simulink model "lab2_task3"  (R2020a)
settings: Solver=FixedStepDiscrete  StartTime=0.0  StopTime=inf  FixedStep=0.02  RelTol=1e-3  EnableMultiTasking=on
values from neighbouring files (symbols this model uses):
  lim = length(xx)    [lab2_task3_4_trajectories.m]
  tt = zeros(size(xx))    [lab2_task3_4_trajectories.m]
  xx = 0:0.5:2*3.14    [lab2_task3_4_trajectories.m]
  yy = sin(0:0.5:2*3.14)    [lab2_task3_4_trajectories.m]
undefined symbols (not defined in the file or in its folder): angdiff, Angular, Linear
libraries: robotlib x3, simulink x2, robotcorelib x1, simulink_extras x1
settings Model: Creator=The MathWorks, Inc.  LastModifiedBy=Pablo
settings DataIOCC: LimitDataPoints=on  SaveFormat=Array  ReturnWorkspaceOutputs=off
settings OptimizationCC: ZeroExternalMemoryAtStartup=off  ZeroInternalMemoryAtStartup=off  LifeSpan=Inf  MaxStackSize=64
settings DebuggingCC: SolverPrmCheckMsg=warning  AllowSymbolicDim=off  SFUnexpectedBacktrackingDiag=warning  SFNoUnconditionalDefaultTransitionDiag=warning  SFExecutionAtInitializationDiag=none  ArithmeticOperatorsInVariantConditions=warning
settings HardwareCC: ProdBitPerPointer=32  ProdBitPerSizeT=32  ProdBitPerPtrDiffT=32  ProdLargestAtomicFloat=None  ProdIntDivRoundTo=Undefined  ProdEndianess=Unspecified  ProdWordSize=32  ProdHWDeviceType=Generic->Unspecified (assume 32-bit Generic)  TargetHWDeviceType=Generic->Unspecified (assume 32-bit Generic)  UseEmbeddedCoderFeatures=off
settings ModelReferenceCC: PropagateSignalLabelsOutOfModel=off
settings SFSimCC: SimUseLocalCustomCode=off  CustomCodeUndefinedFunction=UseInterfaceOnly
settings RTWCC: SystemTargetFile=ert.tlc  HardwareBoard=Robot Operating System (ROS)  TemplateMakefile=ert_default_tmf  RTWUseLocalCustomCode=off  Toolchain=Catkin  TargetLang=C++
settings CodeAppCC: StateflowObjectComments=on
settings ERTTargetCC: MultiwordLength=2048  ERTCustomFileBanners=off  MultiInstanceERTCode=on  CodeInterfacePackaging=C++ class  SupportContinuousTime=on  SupportNonInlinedSFcns=on  RemoveResetFunc=off  SupportVariableSizeSignals=on  ModelStepFunctionPrototypeControlCompliant=off  RootIOFormat=Structure reference  ConvertIfToSwitch=off  SuppressUnreachableDefaultCases=off
settings ConfigComp: CovMetricSettings=dw  CovHtmlReporting=on  CovSaveCumulativeToWorkspaceVar=on  CovSaveSingleToWorkspaceVar=on  CovExternalEMLEnable=off  CovSFcnEnable=off

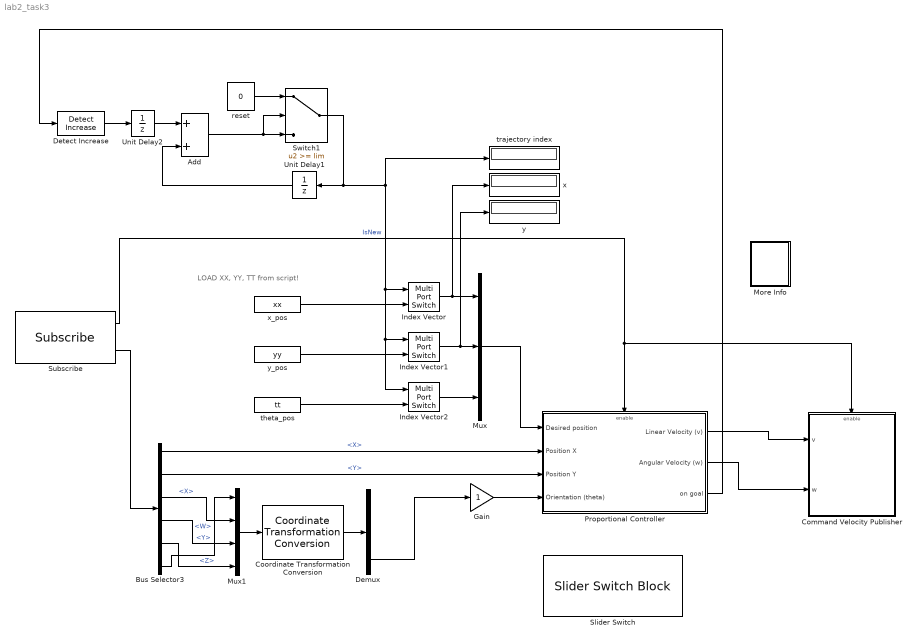
== system lab2_task3 ==
  note: LOAD XX, YY, TT from script!
  Add : Sum
  Bus Selector3 : BusSelector  OutputSignals=Pose.Pose.Position.X,Pose.Pose.Position.Y,Pose.Pose.Orientation.X,Pose.Pose.Orientation.Y,Pose.Pose.Orientation.Z,Pose.Pose.Orientation.W
  Command Velocity Publisher : Subsystem
  Coordinate Transformation Conversion : robotcorelib/Coordinate Transformation Conversion  InputRepresentation=Quaternion  InputEulerSequence=XYZ  ShowTrVecInputPort=on  OutputRepresentation=Euler Angles  OutputEulerSequence=XYZ  ShowTrVecOutputPort=on  SimulateUsing=Interpreted execution
      settings: SourceProductBaseCode=NV,RO,RR
  Demux : Demux  Outputs=3
  Detect Increase : simulink/Logic and Bit Operations/Detect Increase  vinit=0.0  OutDataTypeStr=boolean
  Gain : Gain
  Index Vector : MultiPortSwitch  DataPortOrder=Zero-based contiguous  Inputs=1  zeroidx=on
  Index Vector1 : MultiPortSwitch  DataPortOrder=Zero-based contiguous  Inputs=1  zeroidx=on
  Index Vector2 : MultiPortSwitch  DataPortOrder=Zero-based contiguous  Inputs=1  zeroidx=on
  More Info : Subsystem
      settings: OpenFcn=showdemo(bdroot(gcb))
      mask Display: disp('?')
  Mux : Mux  Inputs=3
  Mux1 : Mux
  Proportional Controller : Subsystem
  Slider Switch : SliderSwitchBlock
      settings: Values={{'STOP OFF', 'STOP ON'}, [0 1]}
  Subscribe : robotlib/Subscribe  topicSource=Select from ROS network  topic=/odom  messageType=nav_msgs/Odometry  sampleTime=-1  messageQueueLength=51
  Switch1 : Switch  Threshold=lim
  Unit Delay1 : UnitDelay  SampleTime=-1  HasFrameUpgradeWarning=on
  Unit Delay2 : UnitDelay  SampleTime=-1  HasFrameUpgradeWarning=on
  reset : Constant  Value=0  VectorParams1D=off
  theta_pos : Constant  Value=tt  VectorParams1D=off
  trajectory index : Display
  x : Display
  x_pos : Constant  Value=xx  VectorParams1D=off
  y : Display
  y_pos : Constant  Value=yy  VectorParams1D=off
  wires:
  Subscribe/2 -> Bus Selector3/1
  Subscribe/1 -> Command Velocity Publisher/Enable, Proportional Controller/Enable  "IsNew"
  Mux/1 -> Proportional Controller/1(Desired position)
  Mux1/1 -> Coordinate Transformation Conversion/1
  Coordinate Transformation Conversion/1 -> Demux/1
  Proportional Controller/2(Angular Velocity (w)) -> Command Velocity Publisher/2(w)
  Proportional Controller/1(Linear Velocity (v)) -> Command Velocity Publisher/1(v)
  Bus Selector3/1 -> Proportional Controller/2(Position X)  "<X>"
  Bus Selector3/2 -> Proportional Controller/3(Position Y)  "<Y>"
  Gain/1 -> Proportional Controller/4(Orientation (theta))
  Bus Selector3/3 -> Mux1/2  "<X>"
  Bus Selector3/4 -> Mux1/3  "<Y>"
  Bus Selector3/5 -> Mux1/4  "<Z>"
  Bus Selector3/6 -> Mux1/1  "<W>"
  Demux/3 -> Gain/1
  Add/1 -> Switch1/2, Switch1/3
  Unit Delay1/1 -> Add/2
  reset/1 -> Switch1/1
  Index Vector2/1 -> Mux/3
  Index Vector1/1 -> y/1, Mux/2
  Index Vector/1 -> Mux/1, x/1
  x_pos/1 -> Index Vector/2
  y_pos/1 -> Index Vector1/2
  theta_pos/1 -> Index Vector2/2
  Proportional Controller/3(on goal) -> Detect Increase/1
  Detect Increase/1 -> Unit Delay2/1
  Unit Delay2/1 -> Add/1
  Switch1/1 -> trajectory index/1, Index Vector1/1, Index Vector2/1, Index Vector/1, Unit Delay1/1

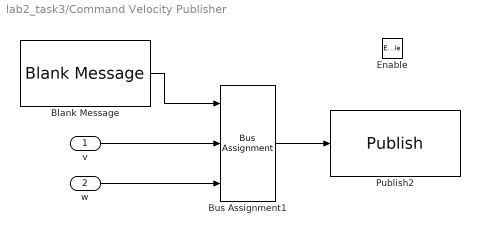
== system lab2_task3/Command Velocity Publisher ==
  v : Inport
  w : Inport  Port=2
  Enable : EnablePort
  Blank Message : robotlib/Blank Message  messageClass=Message  entityType=geometry_msgs/Twist  messageType=geometry_msgs/Twist  SampleTime=inf
  Bus Assignment1 : BusAssignment  DialogController=Simulink.DDGSource_BusAssignment  AssignedSignals=Linear.X,Angular.Z
  Publish2 : robotlib/Publish  topicSource=Select from ROS network  topic=/cmd_vel  messageType=geometry_msgs/Twist  messageQueueLength=105
  wires:
  Bus Assignment1/1 -> Publish2/1
  Blank Message/1 -> Bus Assignment1/1
  v/1 -> Bus Assignment1/2
  w/1 -> Bus Assignment1/3

== system lab2_task3/More Info ==

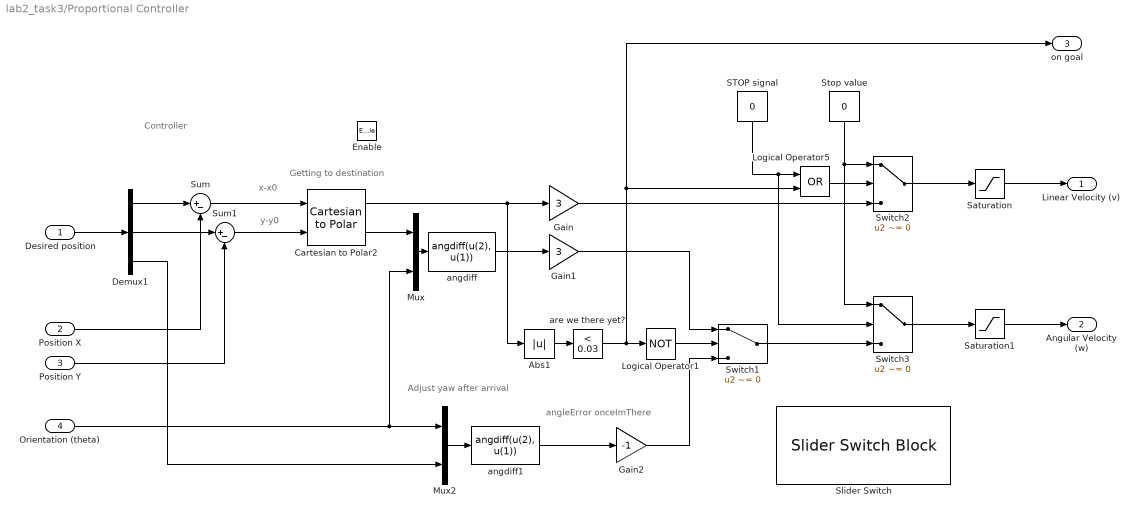
== system lab2_task3/Proportional Controller ==
  note: Adjust yaw after arrival
  note: angleError
      | onceImThere
  note: x-x0
  note: y-y0
  note: Controller
  note: Getting to destination
  Desired position : Inport
  Position X : Inport  Port=2
  Position Y : Inport  Port=3
  Orientation (theta) : Inport  Port=4
  Enable : EnablePort
  Abs1 : Abs
  Cartesian to Polar2 : simulink_extras/Transformations/Cartesian to Polar
  Demux1 : Demux  Outputs=3
  Gain : Gain  Gain=3
  Gain1 : Gain  Gain=3
  Gain2 : Gain  Gain=-1
  Logical Operator1 : Logic  Operator=NOT  AllPortsSameDT=off  OutDataTypeStr=boolean
  Logical Operator5 : Logic  Operator=OR  AllPortsSameDT=off  OutDataTypeStr=boolean
  Mux : Mux  Inputs=2
  Mux2 : Mux  Inputs=2
  STOP signal : Constant  Value=0
  Saturation : Saturate  UpperLimit=0.3  LowerLimit=-0.3  LinearizeAsGain=off
  Saturation1 : Saturate  UpperLimit=999  LowerLimit=-999  LinearizeAsGain=off
  Slider Switch : SliderSwitchBlock
      settings: Values={{'STOP OFF', 'STOP ON'}, [0 1]}
  Stop value : Constant  Value=0
  Sum : Sum  Inputs=|+-
  Sum1 : Sum  Inputs=|+-
  Switch1 : Switch  Criteria=u2 ~= 0
  Switch2 : Switch  Criteria=u2 ~= 0
  Switch3 : Switch  Criteria=u2 ~= 0
  angdiff : MATLABFcn  MATLABFcn=angdiff(u(2), u(1))  OutputDimensions=1  Output1D=off
  angdiff1 : MATLABFcn  MATLABFcn=angdiff(u(2), u(1))  OutputDimensions=1  Output1D=off
  are we there yet? : simulink/Logic and Bit Operations/Compare To Constant  relop=<  const=0.03  OutDataTypeStr=boolean
  Linear Velocity (v) : Outport  VectorParamsAs1DForOutWhenUnconnected=off
  Angular Velocity (w) : Outport  Port=2  VectorParamsAs1DForOutWhenUnconnected=off
  on goal : Outport  Port=3  VectorParamsAs1DForOutWhenUnconnected=off
  wires:
  Stop value/1 -> Switch2/1, Switch3/1
  STOP signal/1 -> Switch3/2, Logical Operator5/1
  Demux1/1 -> Sum/1
  Demux1/2 -> Sum1/1
  Position Y/1 -> Sum1/2
  Position X/1 -> Sum/2
  Sum/1 -> Cartesian to Polar2/1
  Sum1/1 -> Cartesian to Polar2/2
  Cartesian to Polar2/1 -> Gain/1, Abs1/1
  angdiff/1 -> Gain1/1
  Orientation (theta)/1 -> Mux/2, Mux2/1
  Gain/1 -> Switch2/3
  Mux/1 -> angdiff/1
  Saturation/1 -> Linear Velocity (v)/1
  Switch2/1 -> Saturation/1
  Switch3/1 -> Saturation1/1
  Saturation1/1 -> Angular Velocity (w)/1
  Cartesian to Polar2/2 -> Mux/1
  Desired position/1 -> Demux1/1
  Abs1/1 -> are we there yet?/1
  angdiff1/1 -> Gain2/1
  Mux2/1 -> angdiff1/1
  Demux1/3 -> Mux2/2
  Gain2/1 -> Switch1/3
  Gain1/1 -> Switch1/1
  Switch1/1 -> Switch3/3
  are we there yet?/1 -> Logical Operator1/1, Logical Operator5/2, on goal/1
  Logical Operator1/1 -> Switch1/2
  Logical Operator5/1 -> Switch2/2
